simulink model "serial_write_example"  (R2019a)
settings: Solver=ode2  StartTime=0.0  StopTime=inf  FixedStep=0.001  RelTol=1e-3  EnableMultiTasking=on
InitFcn:
  | set_param(gcs, 'ZoomFactor','FitSystem')
model workspace (MAT data in the model file):
  target_system = 1
undefined symbols (not defined in the file or in its folder): HIL
libraries: quarc_library x7, simulink x2
settings Model: SimulationMode=external  ExtModeTrigDuration=10000  Creator=dmadill  LastModifiedBy=user
settings SolverCC: PositivePriorityOrder=on
settings DataIOCC: LimitDataPoints=on  SaveFormat=Array  ReturnWorkspaceOutputs=off
settings OptimizationCC: LifeSpan=inf
settings DebuggingCC: SolverPrmCheckMsg=warning  SFUnexpectedBacktrackingDiag=warning  SFNoUnconditionalDefaultTransitionDiag=warning  SFExecutionAtInitializationDiag=none  ArithmeticOperatorsInVariantConditions=warning
settings HardwareCC: ProdBitPerLong=64  ProdLargestAtomicFloat=None  ProdHWDeviceType=Intel->x86-64
settings ModelReferenceCC: PropagateSignalLabelsOutOfModel=off
settings SFSimCC: SimUseLocalCustomCode=off
settings RTWCC: SystemTargetFile=quarc_linux_x64.tlc  TemplateMakefile=quarc_linux_x64_tmf  Description=QUARC Linux x64 Target  RTWUseLocalCustomCode=off
settings CodeAppCC: StateflowObjectComments=on
settings STFCustomTargetCC: TargetLibSuffix=.a  TargetPreCompLibLocation=C:\PROGRA~3\QUARC\lib\2019a\LINUX_~1\release  ConcurrentExecutionCompliant=on  SystemTargetFile=quarc_linux_x64.tlc
settings GRTTargetCC: TargetLibSuffix=.a  TargetPreCompLibLocation=C:\PROGRA~3\QUARC\lib\2019a\LINUX_~1\release  TargetLangStandard=C89/C90 (ANSI)  ParMdlRefBuildCompliant=off  CompOptLevelCompliant=off  CombineOutputUpdateFcns=off  MatFileLogging=off  CPPClassGenCompliant=off  GRTInterface=on  UseToolchainInfoCompliant=off  ExtMode=on  ExtModeMexFile=quarc_comm  ExtModeMexArgs='-w -d /tmp -uri %u','tcpip://192.168.1.25:17001?retries=10'
settings ConfigComp: CovMetricSettings=dw  CovHtmlReporting=on  CovSaveCumulativeToWorkspaceVar=on  CovSaveSingleToWorkspaceVar=on  CovExternalEMLEnable=off  CovSFcnEnable=off

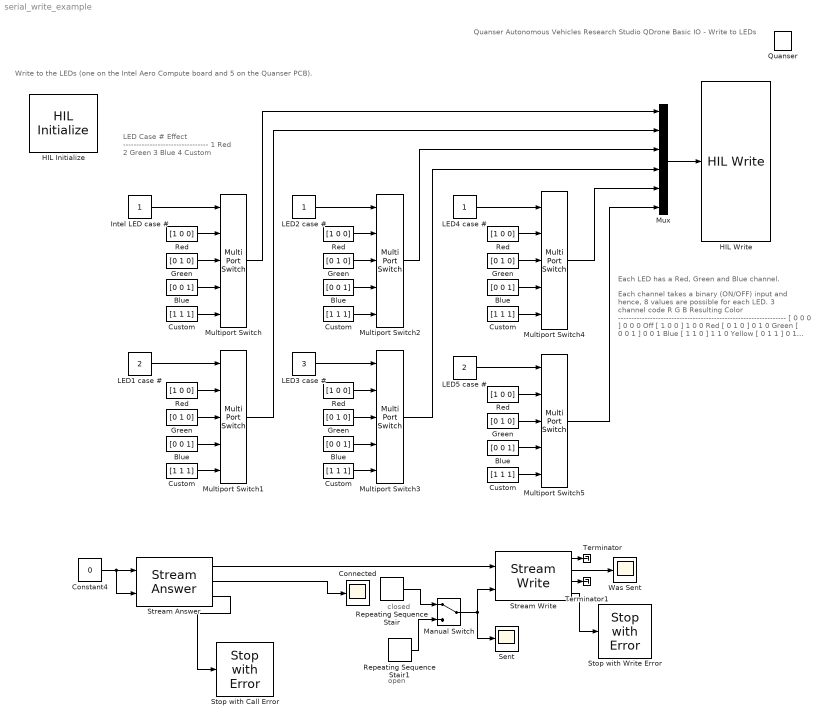
== system serial_write_example ==
  note: closed
  note: open
  note: LED Case # 		Effect
      | --------------------------------
      | 	1			Red
      | 	2			Green
      | 	3			Blue
      | 	4			Custom
  note: Each LED has a Red, Green and Blue channel.
  note: Write to the LEDs (one on the Intel Aero Compute board and 5 on the Quanser PCB).
  note: Quanser Autonomous Vehicles Research Studio
      | QDrone Basic IO - Write to LEDs
  note: Each channel takes a binary (ON/OFF) input and hence, 8 values are possible for each LED.
      |
      | 3 channel code	R	G	B	Resulting Color
      | ---------------------------------------------------------------
      | [ 0  0  0 ]			0	0	0	Off
      | [ 1  0  0 ]			1	0	0	Red
      | [ 0  1  0 ]			0	1	0	Green
      | [ 0  0  1 ]			0	0	1	Blue
      | [ 1  1  0 ]			1	1	0	Yellow
      | [ 0  1  1 ]			0	1	1	Cyan
      | [ 1  0  1 ]			1	0	1	Purple
      | [ 1  1  1 ]			1	1	1	White
  "     Blue     " : Constant  Value=[0 0 1]
  "     Custom     " : Constant  Value=[1 1 1]
  "     Green     " : Constant  Value=[0 1 0]
  "     Red     " : Constant  Value=[1 0 0]
  "    Blue    " : Constant  Value=[0 0 1]
  "    Custom    " : Constant  Value=[1 1 1]
  "    Green    " : Constant  Value=[0 1 0]
  "    Red    " : Constant  Value=[1 0 0]
  "   Blue   " : Constant  Value=[0 0 1]
  "   Custom   " : Constant  Value=[1 1 1]
  "   Green   " : Constant  Value=[0 1 0]
  "   Red   " : Constant  Value=[1 0 0]
  "  Blue  " : Constant  Value=[0 0 1]
  "  Custom  " : Constant  Value=[1 1 1]
  "  Green  " : Constant  Value=[0 1 0]
  "  Red  " : Constant  Value=[1 0 0]
  " Blue " : Constant  Value=[0 0 1]
  " Custom " : Constant  Value=[1 1 1]
  " Green " : Constant  Value=[0 1 0]
  " Red " : Constant  Value=[1 0 0]
  Blue : Constant  Value=[0 0 1]
  Connected : Scope
  Constant4 : Constant  Value=0
  Custom : Constant  Value=[1 1 1]
  Green : Constant  Value=[0 1 0]
  HIL Initialize : quarc_library/Data Acquisition/Generic/Configuration/HIL Initialize  object_name=HIL-1  board_type=qdrone  board_number=0  board_options=gyro_fs=2000;gyro_rate=1000;gyro_os=4;accel_fs=16;accel_rate=400;accel_os=4;baro_os=4096  exclusive=off  active=on  hardware_clocks=[]  clock_modes=[]  initial_clock_frequencies=[]  set_clock_params_at_start=off  set_clock_params_at_switch_in=off  set_clock_frequencies_at_start=off  set_clock_frequencies_at_switch_in=off  analog_input_channels=[0:4]  analog_input_configurations=[]  analog_input_maximums=[3.3]  analog_input_minimums=[0]  set_analog_input_params_at_start=off  set_analog_input_params_at_switch_in=off  analog_output_channels=[]  analog_output_maximums=[]  analog_output_minimums=[]  initial_analog_outputs=[]  final_analog_outputs=[]  watchdog_analog_outputs=[]  set_analog_output_params_at_start=off  set_analog_output_params_at_switch_in=off  set_analog_outputs_at_start=off  set_analog_outputs_at_switch_in=off  set_analog_outputs_at_terminate=off  set_analog_outputs_at_switch_out=off  set_analog_outputs_on_watchdog=off  digital_input_channels=[]  digital_output_channels=[5:7 9:23]  digital_output_configuration=[]  initial_digital_outputs=[0]  final_digital_outputs=[0]  watchdog_digital_outputs=[]  set_digital_output_params_at_start=off  set_digital_output_params_at_switch_in=off  set_digital_outputs_at_start=on  set_digital_outputs_at_switch_in=off  set_digital_outputs_at_terminate=on  set_digital_outputs_at_switch_out=off  set_digital_outputs_on_watchdog=off  encoder_channels=[0:2]  quadrature=[4]  encoder_filter_frequency=50e6/1  initial_encoder_counts=[0]  set_encoder_params_at_start=on  set_encoder_params_at_switch_in=off  set_encoder_counts_at_start=on  set_encoder_counts_at_switch_in=off  pwm_channels=[0:3]  pwm_modes=[4]  pwm_frequency=2000  pwm_configuration=[0]  pwm_alignment=[0]  pwm_polarity=[1]  pwm_leading_deadband=[]  pwm_trailing_deadband=[]  initial_pwm_outputs=[0]  final_pwm_outputs=[0]  watchdog_pwm_outputs=[0]  set_pwm_params_at_start=on  set_pwm_params_at_switch_in=off  set_pwm_outputs_at_start=on  set_pwm_outputs_at_switch_in=off  set_pwm_outputs_at_terminate=on  set_pwm_outputs_at_switch_out=off  set_pwm_outputs_on_watchdog=off  other_output_channels=[]  initial_other_outputs=[]  final_other_outputs=[]  watchdog_other_outputs=[]  set_other_outputs_at_start=off  set_other_outputs_at_switch_in=off  set_other_outputs_at_terminate=off  set_other_outputs_at_switch_out=off  set_other_outputs_on_watchdog=off
      settings: SourceProductName=The database C:\Users\user\AppData\Roaming\MathWorks\MATLAB\R2017a\slblocks_master.db is locked, or a table in the database is locked. (database is locked)
  HIL Write : quarc_library/Data Acquisition/Generic/Immediate I//O/HIL Write  object_name=HIL-1  analog_channels=[]  pwm_channels=[]  digital_channels=[5:7 9:23]  other_channels=[]  sample_time=-1  active=off  vector_input=on
      settings: SourceProductName=The database C:\Users\user\AppData\Roaming\MathWorks\MATLAB\R2017a\slblocks_master.db is locked, or a table in the database is locked. (database is locked)
  Intel LED case # : Constant
  LED1 case # : Constant  Value=2
  LED2 case # : Constant
  LED3 case # : Constant  Value=3
  LED4 case # : Constant
  LED5 case # : Constant  Value=2
  Manual Switch : ManualSwitch
  Multiport Switch{,1..5} (6 alike) : MultiPortSwitch  Inputs=4
  Mux : Mux  Inputs=6
  Quanser : quarc_library/Logos/Quanser
  Red : Constant  Value=[1 0 0]
  Repeating Sequence Stair : simulink/Sources/Repeating Sequence Stair  OutValues=[255 255 1 7 3 30 0 0 0 0 214].'  tsamp=-1  OutMin=[0]  OutMax=[]  OutDataTypeStr=fixdt(0,8,0)  OutputDataTypeScalingMode=Specify via dialog  OutDataType=fixdt(0,8,0)  ConRadixGroup=Best Precision: Vector-wise  OutScaling=[]
  Repeating Sequence Stair1 : simulink/Sources/Repeating Sequence Stair  OutValues=[255 255 1 7 3 30 32 3 0 0 179].'  tsamp=-1  OutMin=[0]  OutMax=[]  OutDataTypeStr=fixdt(0,8,0)  OutputDataTypeScalingMode=Specify via dialog  OutDataType=fixdt(0,8,0)  ConRadixGroup=Best Precision: Vector-wise  OutScaling=[]
  Sent : Scope
  Stop with Call Error : quarc_library/Sinks/Error Handling/Stop with Error  message_type=Interpret input as error code  message=Error occurred
      settings: SourceProductName=QUARC Targets
  Stop with Write Error : quarc_library/Sinks/Error Handling/Stop with Error  message_type=Interpret input as error code  message=Error occurred
      settings: SourceProductName=QUARC Targets
  Stream Answer : quarc_library/Communications/Intermediate/Stream Answer  uri_source=Specify via dialog (do not evaluate)  uri=serial://localhost:1?sndsize='16',baud='9600',word='8'  apply_uri_to_all_configs=on  send_buffer_size=128  receive_buffer_size=128  byte_order=little endian (Intel - LSB first)  sample_time=qc_get_step_size  active=off
      settings: AttributesFormatString="\"serial://localhost:1?sndsize='16',baud='9600',word='8'\""  SourceProductName=QUARC Targets
  Stream Write : quarc_library/Communications/Intermediate/Stream Write  optimization=Minimizing latency  send_dims=off
      settings: SourceProductName=QUARC Targets
  Terminator : Terminator
  Terminator1 : Terminator
  Was Sent : Scope
  wires:
  Blue/1 -> Multiport Switch/4
  Green/1 -> Multiport Switch/3
  Red/1 -> Multiport Switch/2
  "     Red     "/1 -> Multiport Switch1/2
  "     Green     "/1 -> Multiport Switch1/3
  "     Blue     "/1 -> Multiport Switch1/4
  "    Blue    "/1 -> Multiport Switch2/4
  "    Green    "/1 -> Multiport Switch2/3
  "    Red    "/1 -> Multiport Switch2/2
  "   Red   "/1 -> Multiport Switch3/2
  "   Green   "/1 -> Multiport Switch3/3
  "   Blue   "/1 -> Multiport Switch3/4
  "  Blue  "/1 -> Multiport Switch5/4
  "  Green  "/1 -> Multiport Switch5/3
  "  Red  "/1 -> Multiport Switch5/2
  " Red "/1 -> Multiport Switch4/2
  " Green "/1 -> Multiport Switch4/3
  " Blue "/1 -> Multiport Switch4/4
  Intel LED case #/1 -> Multiport Switch/1
  LED1 case #/1 -> Multiport Switch1/1
  LED2 case #/1 -> Multiport Switch2/1
  LED3 case #/1 -> Multiport Switch3/1
  LED4 case #/1 -> Multiport Switch4/1
  LED5 case #/1 -> Multiport Switch5/1
  Multiport Switch/1 -> Mux/1
  Multiport Switch1/1 -> Mux/2
  Multiport Switch2/1 -> Mux/3
  Multiport Switch3/1 -> Mux/4
  Multiport Switch4/1 -> Mux/5
  Multiport Switch5/1 -> Mux/6
  Mux/1 -> HIL Write/1
  Custom/1 -> Multiport Switch/5
  " Custom "/1 -> Multiport Switch1/5
  "  Custom  "/1 -> Multiport Switch3/5
  "   Custom   "/1 -> Multiport Switch2/5
  "    Custom    "/1 -> Multiport Switch4/5
  "     Custom     "/1 -> Multiport Switch5/5
  Stream Write/1 -> Terminator/1
  Stream Answer/3 -> Stop with Call Error/1
  Stream Answer/1 -> Stream Write/1
  Stream Answer/2 -> Connected/1
  Constant4/1 -> Stream Answer/1, Stream Answer/2
  Stream Write/2 -> Was Sent/1
  Stream Write/3 -> Terminator1/1
  Stream Write/4 -> Stop with Write Error/1
  Repeating Sequence Stair1/1 -> Manual Switch/2
  Repeating Sequence Stair/1 -> Manual Switch/1
  Manual Switch/1 -> Stream Write/2, Sent/1
